simulink model "mx1701_3"  (Simulink 8.8)
settings: Solver=VariableStepAuto  StartTime=0.0  StopTime=10.0  RelTol=1e-3
settings Model: SuppressorTable=22 serialization::archive 11 0 3 0 0 0 0 0  Creator=guoshaopan  LastModifiedBy=guoshaopan
settings DataIOCC: LimitDataPoints=off  SaveFormat=Dataset  SignalLoggingSaveFormat=Dataset
settings OptimizationCC: LifeSpan=auto
settings DebuggingCC: UnderspecifiedInitializationDetection=Simplified  MergeDetectMultiDrivingBlocksExec=error  FcnCallInpInsideContextMsg=error  StateNameClashWarn=none  SFUnexpectedBacktrackingDiag=error  SFNoUnconditionalDefaultTransitionDiag=error  SFExecutionAtInitializationDiag=warning
settings HardwareCC: ProdBitPerPointer=64  ProdBitPerSizeT=64  ProdBitPerPtrDiffT=64  ProdLargestAtomicFloat=Float  ProdIntDivRoundTo=Zero  ProdEndianess=LittleEndian  ProdWordSize=64  ProdHWDeviceType=Intel->x86-64 (Windows64)
settings ModelReferenceCC: PropagateSignalLabelsOutOfModel=on
settings GRTTargetCC: TargetLangStandard=C99 (ISO)  GeneratePreprocessorConditionals=Use local settings  CombineOutputUpdateFcns=on  GRTInterface=off
settings ConfigComp: CovMetricSettings=dwe  CovHtmlReporting=off  CovSaveCumulativeToWorkspaceVar=off  CovSaveSingleToWorkspaceVar=off  CovExternalEMLEnable=on

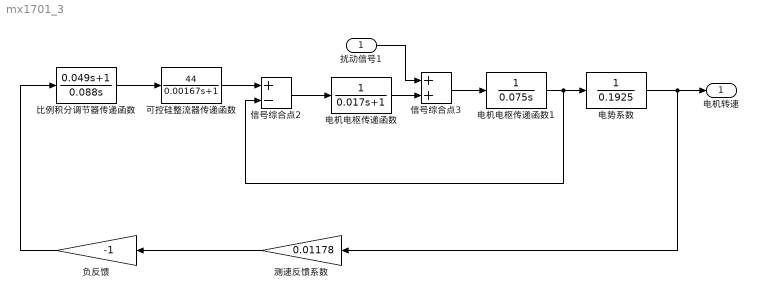
== system mx1701_3 ==
  扰动信号1 : Inport
  " 可控硅整流器传递函数" : TransferFcn  Numerator=[44]  Denominator=[0.00167 1]
  " 电势系数" : TransferFcn  Denominator=[0.1925]
  " 电机电枢传递函数" : TransferFcn  Denominator=[0.017 1]
  " 电机电枢传递函数1" : TransferFcn  Denominator=[0.075 0]
  信号综合点2 : Sum  Inputs=+-
  信号综合点3 : Sum
  比例积分调节器传递函数 : TransferFcn  Numerator=[0.049 1]  Denominator=[0.088 0]
  测速反馈系数 : Gain  Gain=0.01178
  "负反馈 " : Gain  Gain=-1
  电机转速 : Outport
  wires:
  比例积分调节器传递函数/1 -> " 可控硅整流器传递函数"/1
  信号综合点2/1 -> " 电机电枢传递函数"/1
  " 可控硅整流器传递函数"/1 -> 信号综合点2/1
  " 电机电枢传递函数"/1 -> 信号综合点3/2
  扰动信号1/1 -> 信号综合点3/1
  信号综合点3/1 -> " 电机电枢传递函数1"/1
  " 电机电枢传递函数1"/1 -> 信号综合点2/2, " 电势系数"/1
  " 电势系数"/1 -> 测速反馈系数/1, 电机转速/1
  测速反馈系数/1 -> "负反馈 "/1
  "负反馈 "/1 -> 比例积分调节器传递函数/1
